simulink model "LdDblSlave_Runner"  (R2020b)
settings: configuration reference "VLS_Standard_Configuration" (kept outside this file)
undefined symbols (not defined in the file): C_CieCurveGammaToPwmY, C_CieCurvePwmToGammaY, C_DblLeftAngles, C_DblRampTime, C_DblRightAngles, C_DblSlavePeriod, C_EndIndexOfEachLightingModule, C_IsDblActive, C_LedCenterLimits, C_StartIndexOfEachLightingModule
libraries: DblSlaveLib x1
settings Model: DataDictionary=LdAfsDblSlaveDD_SingleLed.sldd  EnableAccessToBaseWorkspace=off  Creator=ahashem  LastModifiedBy=ahashem
settings ConfigSetRef: SourceName=VLS_Standard_Configuration

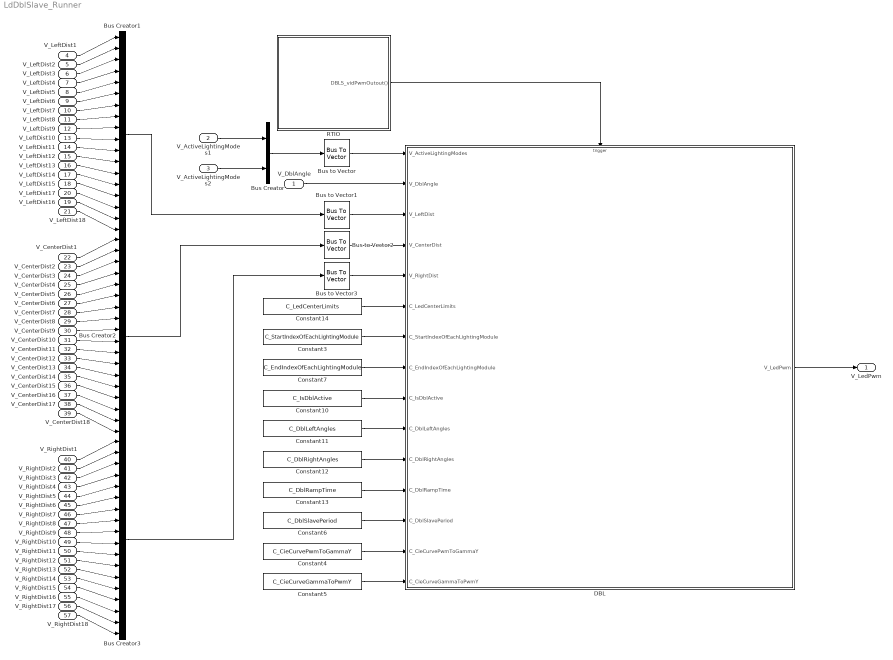
== system LdDblSlave_Runner ==
  V_DblAngle : Inport
  V_ActiveLightingModes1 : Inport  Port=2
  V_ActiveLightingModes2 : Inport  Port=3
  V_LeftDist1 : Inport  Port=4
  V_LeftDist2 : Inport  Port=5
  V_LeftDist3 : Inport  Port=6
  V_LeftDist4 : Inport  Port=7
  V_LeftDist5 : Inport  Port=8
  V_LeftDist6 : Inport  Port=9
  V_LeftDist7 : Inport  Port=10
  V_LeftDist8 : Inport  Port=11
  V_LeftDist9 : Inport  Port=12
  V_LeftDist10 : Inport  Port=13
  V_LeftDist11 : Inport  Port=14
  V_LeftDist12 : Inport  Port=15
  V_LeftDist13 : Inport  Port=16
  V_LeftDist14 : Inport  Port=17
  V_LeftDist15 : Inport  Port=18
  V_LeftDist16 : Inport  Port=19
  V_LeftDist17 : Inport  Port=20
  V_LeftDist18 : Inport  Port=21
  V_CenterDist1 : Inport  Port=22
  V_CenterDist2 : Inport  Port=23
  V_CenterDist3 : Inport  Port=24
  V_CenterDist4 : Inport  Port=25
  V_CenterDist5 : Inport  Port=26
  V_CenterDist6 : Inport  Port=27
  V_CenterDist7 : Inport  Port=28
  V_CenterDist8 : Inport  Port=29
  V_CenterDist9 : Inport  Port=30
  V_CenterDist10 : Inport  Port=31
  V_CenterDist11 : Inport  Port=32
  V_CenterDist12 : Inport  Port=33
  V_CenterDist13 : Inport  Port=34
  V_CenterDist14 : Inport  Port=35
  V_CenterDist15 : Inport  Port=36
  V_CenterDist16 : Inport  Port=37
  V_CenterDist17 : Inport  Port=38
  V_CenterDist18 : Inport  Port=39
  V_RightDist1 : Inport  Port=40
  V_RightDist2 : Inport  Port=41
  V_RightDist3 : Inport  Port=42
  V_RightDist4 : Inport  Port=43
  V_RightDist5 : Inport  Port=44
  V_RightDist6 : Inport  Port=45
  V_RightDist7 : Inport  Port=46
  V_RightDist8 : Inport  Port=47
  V_RightDist9 : Inport  Port=48
  V_RightDist10 : Inport  Port=49
  V_RightDist11 : Inport  Port=50
  V_RightDist12 : Inport  Port=51
  V_RightDist13 : Inport  Port=52
  V_RightDist14 : Inport  Port=53
  V_RightDist15 : Inport  Port=54
  V_RightDist16 : Inport  Port=55
  V_RightDist17 : Inport  Port=56
  V_RightDist18 : Inport  Port=57
  Bus Creator : BusCreator  Inputs=2
  Bus Creator1 : BusCreator  Inputs=18
  Bus Creator2 : BusCreator  Inputs=18
  Bus Creator3 : BusCreator  Inputs=18
  Bus to Vector{,1..3} (4 alike) : BusToVector
  Constant10 : Constant  Value=C_IsDblActive
  Constant11 : Constant  Value=C_DblLeftAngles
  Constant12 : Constant  Value=C_DblRightAngles
  Constant13 : Constant  Value=C_DblRampTime
  Constant14 : Constant  Value=C_LedCenterLimits
  Constant3 : Constant  Value=C_StartIndexOfEachLightingModule
  Constant4 : Constant  Value=C_CieCurvePwmToGammaY
  Constant5 : Constant  Value=C_CieCurveGammaToPwmY
  Constant6 : Constant  Value=C_DblSlavePeriod
  Constant7 : Constant  Value=C_EndIndexOfEachLightingModule
  DBL : Subsystem  Description=Clustering subsystem
  RTIO : Stateflow chart  TreatAsAtomicUnit=on  SystemSampleTime=0.02
  V_LedPwm : Outport  VectorParamsAs1DForOutWhenUnconnected=off
  wires:
  Constant4/1 -> DBL/14(C_CieCurvePwmToGammaY)
  Constant5/1 -> DBL/15(C_CieCurveGammaToPwmY)
  Constant6/1 -> DBL/13(C_DblSlavePeriod)
  Constant10/1 -> DBL/9(C_IsDblActive)
  Constant11/1 -> DBL/10(C_DblLeftAngles)
  Constant12/1 -> DBL/11(C_DblRightAngles)
  V_DblAngle/1 -> DBL/2(V_DblAngle)
  DBL/1(V_LedPwm) -> V_LedPwm/1
  Constant14/1 -> DBL/6(C_LedCenterLimits)
  Constant13/1 -> DBL/12(C_DblRampTime)
  Constant7/1 -> DBL/8(C_EndIndexOfEachLightingModule)
  RTIO/1(DBLS_vidPwmOutout()) -> DBL/Trigger
  Constant3/1 -> DBL/7(C_StartIndexOfEachLightingModule)
  Bus to Vector/1 -> DBL/1(V_ActiveLightingModes)
  Bus Creator/1 -> Bus to Vector/1
  V_ActiveLightingModes2/1 -> Bus Creator/2
  V_ActiveLightingModes1/1 -> Bus Creator/1
  V_LeftDist7/1 -> Bus Creator1/7
  V_LeftDist8/1 -> Bus Creator1/8
  V_LeftDist6/1 -> Bus Creator1/6
  V_LeftDist9/1 -> Bus Creator1/9
  V_LeftDist5/1 -> Bus Creator1/5
  V_LeftDist10/1 -> Bus Creator1/10
  V_LeftDist4/1 -> Bus Creator1/4
  V_LeftDist11/1 -> Bus Creator1/11
  V_LeftDist3/1 -> Bus Creator1/3
  V_LeftDist12/1 -> Bus Creator1/12
  V_LeftDist2/1 -> Bus Creator1/2
  V_LeftDist13/1 -> Bus Creator1/13
  V_LeftDist1/1 -> Bus Creator1/1
  V_LeftDist14/1 -> Bus Creator1/14
  V_LeftDist15/1 -> Bus Creator1/15
  V_LeftDist17/1 -> Bus Creator1/16
  V_LeftDist16/1 -> Bus Creator1/17
  V_LeftDist18/1 -> Bus Creator1/18
  V_CenterDist6/1 -> Bus Creator2/6
  V_CenterDist8/1 -> Bus Creator2/8
  V_CenterDist11/1 -> Bus Creator2/11
  V_CenterDist4/1 -> Bus Creator2/4
  V_CenterDist3/1 -> Bus Creator2/3
  V_CenterDist12/1 -> Bus Creator2/12
  V_CenterDist13/1 -> Bus Creator2/13
  V_CenterDist2/1 -> Bus Creator2/2
  V_CenterDist5/1 -> Bus Creator2/5
  V_CenterDist14/1 -> Bus Creator2/14
  V_CenterDist7/1 -> Bus Creator2/7
  V_CenterDist9/1 -> Bus Creator2/9
  V_CenterDist15/1 -> Bus Creator2/15
  V_CenterDist10/1 -> Bus Creator2/10
  V_CenterDist18/1 -> Bus Creator2/18
  V_CenterDist16/1 -> Bus Creator2/16
  V_CenterDist17/1 -> Bus Creator2/17
  V_CenterDist1/1 -> Bus Creator2/1
  V_RightDist3/1 -> Bus Creator3/3
  V_RightDist17/1 -> Bus Creator3/17
  V_RightDist11/1 -> Bus Creator3/11
  V_RightDist6/1 -> Bus Creator3/6
  V_RightDist8/1 -> Bus Creator3/8
  V_RightDist16/1 -> Bus Creator3/16
  V_RightDist7/1 -> Bus Creator3/7
  V_RightDist14/1 -> Bus Creator3/14
  V_RightDist2/1 -> Bus Creator3/2
  V_RightDist4/1 -> Bus Creator3/4
  V_RightDist5/1 -> Bus Creator3/5
  V_RightDist9/1 -> Bus Creator3/9
  V_RightDist15/1 -> Bus Creator3/15
  V_RightDist18/1 -> Bus Creator3/18
  V_RightDist1/1 -> Bus Creator3/1
  V_RightDist10/1 -> Bus Creator3/10
  V_RightDist13/1 -> Bus Creator3/13
  V_RightDist12/1 -> Bus Creator3/12
  Bus Creator1/1 -> Bus to Vector1/1
  Bus to Vector1/1 -> DBL/3(V_LeftDist)
  Bus Creator2/1 -> Bus to Vector2/1
  Bus to Vector2/1 -> DBL/4(V_CenterDist)
  Bus Creator3/1 -> Bus to Vector3/1
  Bus to Vector3/1 -> DBL/5(V_RightDist)

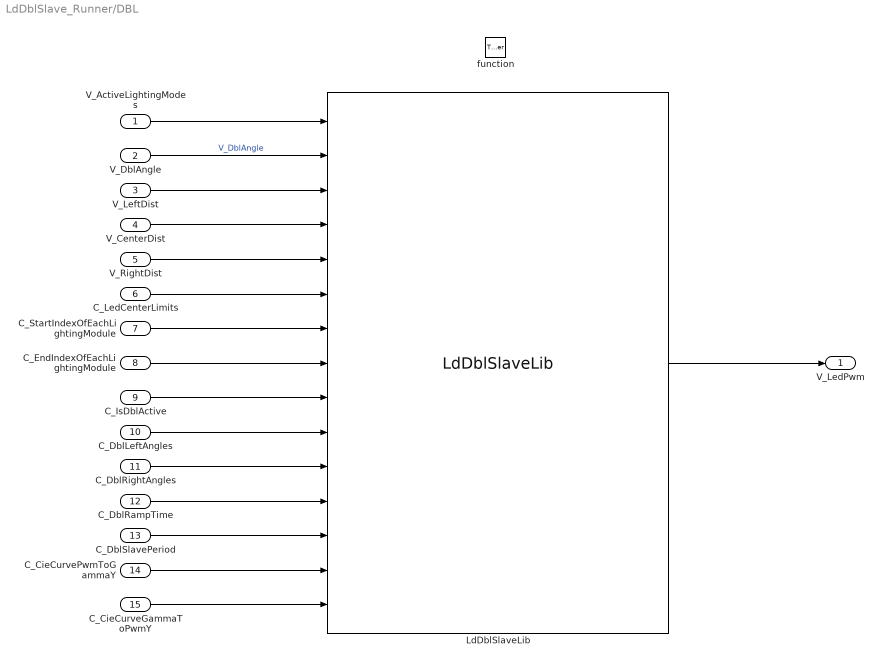
== system LdDblSlave_Runner/DBL ==
  V_ActiveLightingModes : Inport
  V_DblAngle : Inport  Port=2
  V_LeftDist : Inport  Port=3
  V_CenterDist : Inport  Port=4
  V_RightDist : Inport  Port=5
  C_LedCenterLimits : Inport  Port=6
  C_StartIndexOfEachLightingModule : Inport  Port=7
  C_EndIndexOfEachLightingModule : Inport  Port=8
  C_IsDblActive : Inport  Port=9
  C_DblLeftAngles : Inport  Port=10
  C_DblRightAngles : Inport  Port=11
  C_DblRampTime : Inport  Port=12
  C_DblSlavePeriod : Inport  Port=13
  C_CieCurvePwmToGammaY : Inport  Port=14
  C_CieCurveGammaToPwmY : Inport  Port=15
  function : TriggerPort  TriggerType=function-call  VariantControl=Variant
      settings: AttributesFormatString=StatesWhenEnabling: %<StatesWhenEnabling>
  LdDblSlaveLib : DblSlaveLib/LdDblSlaveLib  SystemSampleTime=-1  VariantActivationTime=update diagram  Latency=0  AutoFrameSizeCalculation=off
      link override DblCalc/ActiveModule/DblActive/MultiLed/Selector: IndexMode=One-based
  V_LedPwm : Outport  VectorParamsAs1DForOutWhenUnconnected=off
  wires:
  C_DblRightAngles/1 -> LdDblSlaveLib/11
  C_DblLeftAngles/1 -> LdDblSlaveLib/10
  C_IsDblActive/1 -> LdDblSlaveLib/9
  V_ActiveLightingModes/1 -> LdDblSlaveLib/1
  C_DblRampTime/1 -> LdDblSlaveLib/12
  V_DblAngle/1 -> LdDblSlaveLib/2  "V_DblAngle"
  C_StartIndexOfEachLightingModule/1 -> LdDblSlaveLib/7
  C_LedCenterLimits/1 -> LdDblSlaveLib/6
  V_CenterDist/1 -> LdDblSlaveLib/4
  V_RightDist/1 -> LdDblSlaveLib/5
  V_LeftDist/1 -> LdDblSlaveLib/3
  C_EndIndexOfEachLightingModule/1 -> LdDblSlaveLib/8
  LdDblSlaveLib/1 -> V_LedPwm/1
  C_CieCurvePwmToGammaY/1 -> LdDblSlaveLib/14
  C_DblSlavePeriod/1 -> LdDblSlaveLib/13
  C_CieCurveGammaToPwmY/1 -> LdDblSlaveLib/15

== stateflow chart LdDblSlave_Runner/RTIO ==
  state Schedule
    on every(1,tick):
    send(DBLS_vidPwmOutout);
  (default) -> Schedule
  events: DBLS_vidPwmOutout output FUNCTION_CALL_EVENT
